simulink model "controller"  (R2021b)
settings: Solver=FixedStepAuto  StartTime=0.0  StopTime=10.0  FixedStep=1/10  RelTol=1e-3
settings Model: Creator=DAUIN-Win10  LastModifiedBy=sagai

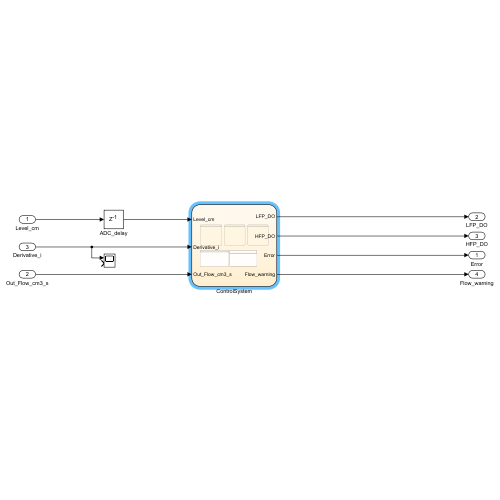
[thumbnail: Simulink's stored preview of the top-level diagram]
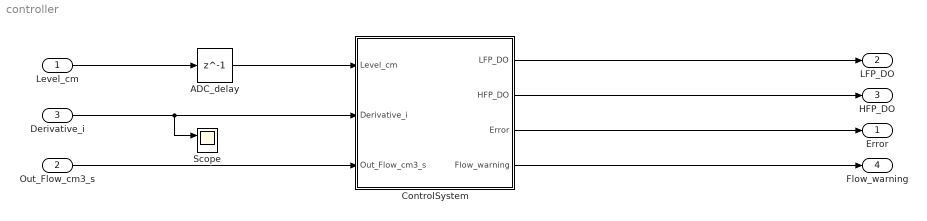
== system controller ==
  Level_cm : Inport
  Out_Flow_cm3_s : Inport  Port=2
  Derivative_i : Inport  Port=3
  ADC_delay : Delay  DelayLength=1  InitialCondition=0
  ControlSystem : Stateflow chart  TreatAsAtomicUnit=on
  Scope : Scope  NumInputPorts=2
  Error : Outport  OutDataTypeStr=boolean
  LFP_DO : Outport  Port=2  OutDataTypeStr=boolean
  HFP_DO : Outport  Port=3  OutDataTypeStr=boolean
  Flow_warning : Outport  Port=4  OutDataTypeStr=boolean
  wires:
  Level_cm/1 -> ADC_delay/1
  ADC_delay/1 -> ControlSystem/1(Level_cm)
  ControlSystem/1(LFP_DO) -> LFP_DO/1
  ControlSystem/2(HFP_DO) -> HFP_DO/1
  ControlSystem/3(Error) -> Error/1
  Derivative_i/1 -> Scope/1, ControlSystem/2(Derivative_i)
  Out_Flow_cm3_s/1 -> ControlSystem/3(Out_Flow_cm3_s)
  ControlSystem/4(Flow_warning) -> Flow_warning/1

== stateflow chart controller/ControlSystem ==
  state PumpLogic [parallel]
    settings: executionOrder=1
    state Off
      en: LFP_DO=0;
      HFP_DO=0;
    state On
      during: PumpTable(Derivative_i, Level_cm);
    (default) -> Off
    Off -> On : [Level_cm<180]
    On -> Off : [Level_cm>180&&Derivative_i>0]
  state ErrorControl [parallel]
    settings: executionOrder=2
    state OK
      en: Error=0;
    state Error
    (default) -> ErrorControl.OK
    ErrorControl.OK -> Error : [Level_cm>200|| Level_cm<0]{Error=1}
    Error -> ErrorControl.OK : [Level_cm<200]
  state PumpControl [parallel]
    settings: executionOrder=3
    state OK
      en:Flow_warning=0;
    state Warning
      en: Flow_warning=1;
    (default) -> PumpControl.OK
    PumpControl.OK -> Warning : [PumpRateFlow(Out_Flow_cm3_s, LFP_DO, HFP_DO) -Derivative_i!=0]
    Warning -> PumpControl.OK : [PumpRateFlow(Out_Flow_cm3_s, LFP_DO, HFP_DO)-Derivative_i==0]
  state PumpTable(i,level) [function]
    (default) -> (junction 61)
    (junction 61) -> (junction 73) : {
        | /* Tank level is decreasing and level_cm is low */
        | aVarTruthTableCondition_1 = (i<0 && level<150);
        | }
    (junction 73) -> (junction 70) : {
        | /* Tank level is decreasing and level_cm is high */
        | aVarTruthTableCondition_2 = (i<0 && (level>=150 && level<175));
        | }
    (junction 70) -> (junction 67) : {
        | /* Tank level is increasing and level_cm is low */
        | aVarTruthTableCondition_3 = (i>0 && level<155);
        | }
    (junction 67) -> (junction 76) : {
        | /* Tank level is increasing and level_cm is high */
        | aVarTruthTableCondition_4 = (i>0 && level>=155);
        | }
    (junction 76) -> (junction 77) [order 1] : [aVarTruthTableCondition_1 && !aVarTruthTableCondition_2 && !aVarTruthTableCondition_3 && !aVarTruthTableCondition_4]
    (junction 77) -> (junction 88) : {
        | /* 'A1':Turn on High Flow Pump */
        | HFP_DO=1; LFP_DO=0;
        | }
    (junction 76) -> (junction 80) [order 2]
    (junction 80) -> (junction 81) [order 1] : [!aVarTruthTableCondition_1 && aVarTruthTableCondition_2 && !aVarTruthTableCondition_3 && !aVarTruthTableCondition_4]
    (junction 81) -> (junction 90) : {
        | /* 'A2':Turn on Low Flow Pump */
        | HFP_DO=0; LFP_DO=1;
        | }
    (junction 80) -> (junction 84) [order 2]
    (junction 84) -> (junction 85) [order 1] : [!aVarTruthTableCondition_1 && !aVarTruthTableCondition_2 && aVarTruthTableCondition_3 && !aVarTruthTableCondition_4]
    (junction 85) -> (junction 92) : {
        | /* 'A1':Turn on High Flow Pump */
        | HFP_DO=1; LFP_DO=0;
        | }
    (junction 84) -> (junction 63) [order 2]
    (junction 63) -> (junction 65) [order 1] : [!aVarTruthTableCondition_1 && !aVarTruthTableCondition_2 && !aVarTruthTableCondition_3 && aVarTruthTableCondition_4]
    (junction 65) -> (junction 94) : {
        | /* 'A2':Turn on Low Flow Pump */
        | HFP_DO=0; LFP_DO=1;
        | }
    (junction 63) -> (junction 107) [order 2]
    (junction 107) -> (junction 109) : /* Default */
    (junction 109) -> (junction 111) : {
        | /* 'A3':Turn off device */
        | HFP_DO=0; LFP_DO=0;
        | }
  data: aVarTruthTableCondition_4 temporary boolean =0; aVarTruthTableCondition_3 temporary boolean =0; aVarTruthTableCondition_2 temporary boolean =0; aVarTruthTableCondition_1 temporary boolean =0; i function_input double; level function_input double; out_flow function_input double; pump_low function_input double; pump_high function_input double; f function_output double; Level_cm input double size=1; LFP_DO output boolean size=1; HFP_DO output boolean size=1; Error output boolean; Derivative_i input double size=1; Out_Flow_cm3_s input double size=1; Flow_warning output boolean size=1
  data aVarTruthTableCondition_4 settings: description=Tank level is increasing and level_cm is high
  data aVarTruthTableCondition_3 settings: description=Tank level is increasing and level_cm is low
  data aVarTruthTableCondition_2 settings: description=Tank level is decreasing and level_cm is high
  data aVarTruthTableCondition_1 settings: description=Tank level is decreasing and level_cm is low
  function f = PumpRateFlow(out_flow, pump_low, pump_high):
    | function f = PumpRateFlow(out_flow, pump_low, pump_high)
    | 
    |     if (pump_low)
    |         f=1-out_flow*0.5;
    | 
    |     elseif(pump_high)
    |         f=3-out_flow*0.5;
    |     
    |     else
    |         f=0-out_flow*0.5;
    |     end
    | end
